simulink model "final_trust"  (R2014b)
settings: Solver=ode45  StartTime=0.0  StopTime=35  RelTol=1e-3
values from neighbouring files (symbols this model uses):
  adapt = 1    [init.m]    (also in init_model.m; init_mussels.m; init_mussels_2.m; init_mussels_konfiguracija_blizu.m)
  delta_0 = zeros(M,M)    [init_model.m]    (also in rander.m = zeros(n,1))
  K = 0.02    [init.m]    (also in init_model.m; init_mussels.m; init_mussels_2.m; init_mussels_konfiguracija_blizu.m)
  ko = ones(n,1)    [rander.m]
  n = input(prompt)    [init.m]    (also in init_consensus.m = 4; init_consensus_15.m = 15; init_mussels.m = 5; init_mussels_2.m = 5)
  sigma_0 = [ 0    0.7   0    0    0 ... (first row only)    [init.m]    (also in init_model.m = zeros(M,M); init_mussels.m = zeros(n,n); init_mussels_2.m; init_mussels_konfiguracija_blizu.m = [ 0    0.7   0.4    0.6    0.5)
  sko_x = transp(sko_x)    [fishplot.m]    (also in rander.m = [0.5, 1.5, 4, 4.5, 5, 7, 8, 9.5])
  sko_y = transp(sko_y)    [fishplot.m]    (also in rander.m = [8, 3, 5, 1, 4.5, 9, 3, 6])
  stream_x = [0.05,0.05,0.05,0.05]    [rander.m]
  stream_y = [0.03,0.03,0.03,0.03]    [rander.m]
  zeta_0 = zeros(n,n)    [init.m]    (also in init_model.m = zeros(M,M); init_mussels.m; init_mussels_2.m; init_mussels_konfiguracija_blizu.m)
undefined symbols (not defined in the file or in its folder): c_0, r, X, Y
settings Model: Creator=Demijan  LastModifiedBy=Demijan

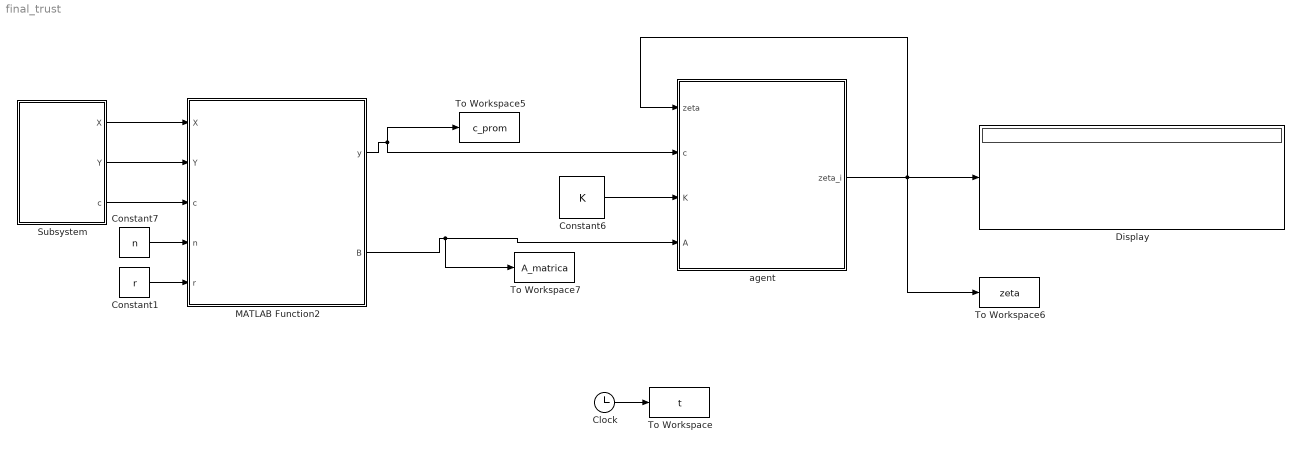
== system final_trust ==
  Clock : Clock
  Constant1 : Constant  Value=r
  Constant6 : Constant  Value=K
  Constant7 : Constant  Value=n
  Display : Display
  MATLAB Function2 : MATLAB Function  TreatAsAtomicUnit=on
  Subsystem : Subsystem
  To Workspace : ToWorkspace  VariableName=t  SampleTime=-1
  To Workspace5 : ToWorkspace  VariableName=c_prom  SampleTime=-1
  To Workspace6 : ToWorkspace  VariableName=zeta  SampleTime=-1
  To Workspace7 : ToWorkspace  VariableName=A_matrica  SampleTime=-1
  "agent " : Subsystem
  wires:
  Constant7/1 -> MATLAB Function2/4(n)
  Subsystem/3(c) -> MATLAB Function2/3(c)
  Subsystem/2(Y) -> MATLAB Function2/2(Y)
  Subsystem/1(X) -> MATLAB Function2/1(X)
  Constant6/1 -> "agent "/3(K)
  MATLAB Function2/1(y) -> "agent "/2(c), To Workspace5/1
  "agent "/1(zeta_i) -> Display/1, "agent "/1(zeta), To Workspace6/1
  Clock/1 -> To Workspace/1
  MATLAB Function2/2(B) -> "agent "/4(A), To Workspace7/1
  Constant1/1 -> MATLAB Function2/5(r)

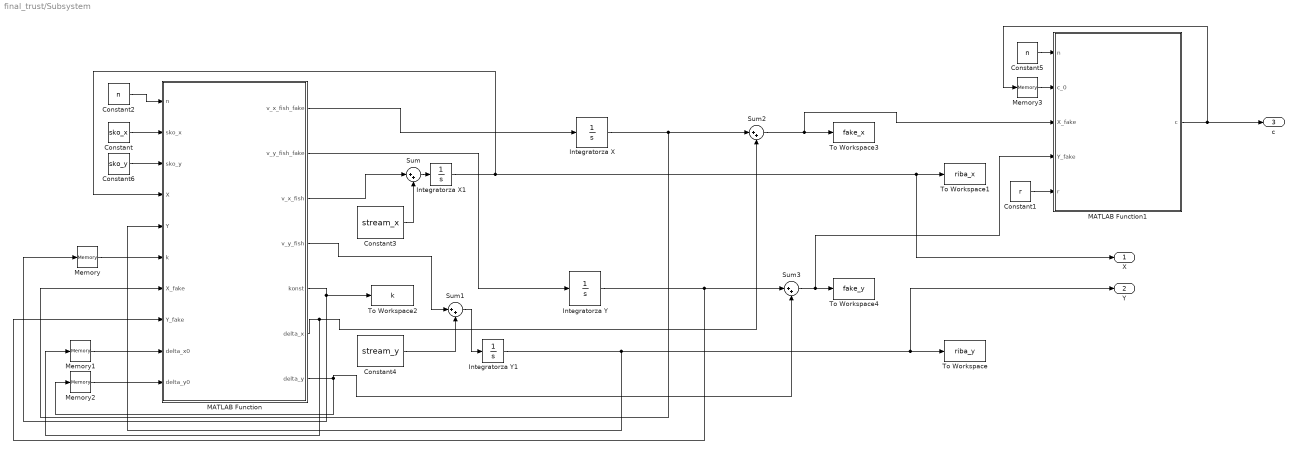
== system final_trust/Subsystem ==
  Constant : Constant  Value=sko_x
  Constant1 : Constant  Value=r
  Constant2 : Constant  Value=n
  Constant3 : Constant  Value=stream_x
  Constant4 : Constant  Value=stream_y
  Constant5 : Constant  Value=n
  Constant6 : Constant  Value=sko_y
  Integratorza X : Integrator  InitialCondition=X  LimitOutput=on  UpperSaturationLimit=10  LowerSaturationLimit=0
  Integratorza X1 : Integrator  InitialCondition=X  LimitOutput=on  UpperSaturationLimit=10  LowerSaturationLimit=0
  Integratorza Y : Integrator  InitialCondition=Y  LimitOutput=on  UpperSaturationLimit=10  LowerSaturationLimit=0
  Integratorza Y1 : Integrator  InitialCondition=Y  LimitOutput=on  UpperSaturationLimit=10  LowerSaturationLimit=0
  MATLAB Function : MATLAB Function  TreatAsAtomicUnit=on
  MATLAB Function1 : MATLAB Function  TreatAsAtomicUnit=on
  Memory : Memory  X0=ko  LinearizeAsDelay=on
  Memory1 : Memory  X0=delta_0  LinearizeAsDelay=on
  Memory2 : Memory  X0=delta_0  LinearizeAsDelay=on
  Memory3 : Memory  X0=c_0  LinearizeAsDelay=on
  Sum{,1..3} (4 alike) : Sum  Inputs=|++
  To Workspace : ToWorkspace  VariableName=riba_y  SaveFormat=Structure With Time  SampleTime=-1
  To Workspace1 : ToWorkspace  VariableName=riba_x  SaveFormat=Structure With Time  SampleTime=-1
  To Workspace2 : ToWorkspace  VariableName=k  SaveFormat=Structure With Time  SampleTime=-1
  To Workspace3 : ToWorkspace  VariableName=fake_x  SampleTime=-1
  To Workspace4 : ToWorkspace  VariableName=fake_y  SampleTime=-1
  X : Outport
  Y : Outport  Port=2
  c : Outport  Port=3
  wires:
  Constant2/1 -> MATLAB Function/1(n)
  Constant6/1 -> MATLAB Function/3(sko_y)
  Constant/1 -> MATLAB Function/2(sko_x)
  MATLAB Function/5(konst) -> To Workspace2/1, Memory/1
  Constant3/1 -> Sum/2
  Sum/1 -> Integratorza X1/1
  Constant4/1 -> Sum1/2
  Sum1/1 -> Integratorza Y1/1
  Integratorza Y1/1 -> MATLAB Function/5(Y), Y/1, To Workspace/1
  Integratorza X1/1 -> To Workspace1/1, X/1, MATLAB Function/4(X)
  Memory/1 -> MATLAB Function/6(k)
  MATLAB Function/6(delta_x) -> Memory1/1, Sum2/2
  MATLAB Function/7(delta_y) -> Sum3/2, Memory2/1
  Integratorza Y/1 -> MATLAB Function/8(Y_fake), Sum3/1
  Integratorza X/1 -> MATLAB Function/7(X_fake), Sum2/1
  Memory2/1 -> MATLAB Function/10(delta_y0)
  Memory1/1 -> MATLAB Function/9(delta_x0)
  MATLAB Function/1(v_x_fish_fake) -> Integratorza X/1
  MATLAB Function/3(v_x_fish) -> Sum/1
  MATLAB Function/4(v_y_fish) -> Sum1/1
  MATLAB Function/2(v_y_fish_fake) -> Integratorza Y/1
  Sum2/1 -> MATLAB Function1/3(X_fake), To Workspace3/1
  Sum3/1 -> MATLAB Function1/4(Y_fake), To Workspace4/1
  Constant1/1 -> MATLAB Function1/5(r)
  Constant5/1 -> MATLAB Function1/1(n)
  Memory3/1 -> MATLAB Function1/2(c_0)
  MATLAB Function1/1(c) -> Memory3/1, c/1

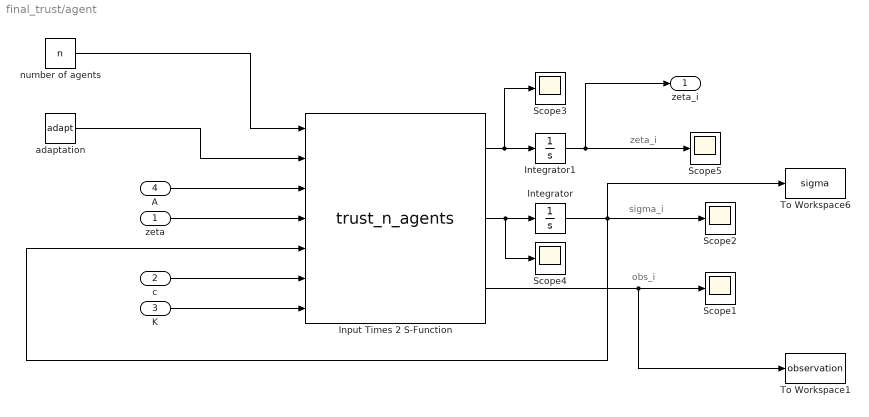
== system final_trust/agent  ==
  note: obs_i
  note: sigma_i
  note: zeta_i
  zeta : Inport
  c : Inport  Port=2
  K : Inport  Port=3
  A : Inport  Port=4
  Input Times 2 S-Function : S-Function  FunctionName=trust_n_agents  EnableBusSupport=off
  Integrator : Integrator  InitialCondition=sigma_0
  Integrator1 : Integrator  InitialCondition=zeta_0
  Scope{1..5} (5 alike) : Scope
      Scope1 settings: TimeRange=20  YMin=0.25  YMax=0.95
      Scope2 settings: TimeRange=20  YMin=0.25  YMax=0.95
      Scope3 settings: TimeRange=20  YMin=0.25  YMax=0.95  SaveName=ScopeData3
      Scope4 settings: TimeRange=20  YMin=0.25  YMax=0.95  SaveName=ScopeData4
      Scope5 settings: TimeRange=20  YMin=0.25  YMax=0.95  SaveName=ScopeData2
  To Workspace1 : ToWorkspace  VariableName=observation  SampleTime=-1
  To Workspace6 : ToWorkspace  VariableName=sigma  SampleTime=-1
  adaptation : Constant  Value=adapt
  number of agents : Constant  Value=n
  zeta_i : Outport
  wires:
  Integrator/1 -> Scope2/1, Input Times 2 S-Function/5, To Workspace6/1
  Integrator1/1 -> zeta_i/1, Scope5/1
  c/1 -> Input Times 2 S-Function/6
  K/1 -> Input Times 2 S-Function/7
  Input Times 2 S-Function/2 -> Scope4/1, Integrator/1
  Input Times 2 S-Function/1 -> Scope3/1, Integrator1/1
  Input Times 2 S-Function/3 -> To Workspace1/1, Scope1/1
  number of agents/1 -> Input Times 2 S-Function/1
  adaptation/1 -> Input Times 2 S-Function/2
  zeta/1 -> Input Times 2 S-Function/4
  A/1 -> Input Times 2 S-Function/3

== matlab function final_trust/MATLAB Function2 ==
  settings: updateMethod=DISCRETE  sampleTime=0.01
  data: y output; X input; Y input; c input; n input; B output; r input
function [y,B] = fish(X, Y, c, n, r)
A=zeros(20,20);
for i=1:n;
    for j=1:n;
        R = sqrt(((X(i)-X(j))^2+(Y(i)-Y(j))^2));
        if R < r && i~=j;
            A(i,j)=1;
        else
            A(i,j)=0;
        end
    end
end
B=zeros(4,4);
for i=1:n;
    for j=1:n;
        B(i,j)=A(i,j);
    end
end
y=zeros(4);
for i=1:n
  for j=1:n
      y(i,j)=A(i,j)*c(i,j);
  end
end

== matlab function final_trust/Subsystem/MATLAB Function ==
  data: v_x_fish_fake output; v_y_fish_fake output; n input; v_x_fish output; sko_x input; sko_y input; v_y_fish output; X input; Y input; k input; X_fake input; konst output; delta_x output; Y_fake input; delta_y output; delta_x0 input; delta_y0 input
function [v_x_fish_fake,v_y_fish_fake,v_x_fish,v_y_fish,konst,delta_x,delta_y] = fcn(n,sko_x, sko_y, X, Y,k,X_fake,Y_fake,delta_x0,delta_y0)
        d=[0; 0; 0; 0; 0; 0; 0; 0];        
        d_fake=[0; 0; 0; 0];
        red=zeros(4,8);
        red(1,:)=[1 3 1 2 3 2 1 3];
        red(2,:)=[2 3 1 3 1 3 1 2];
        red(3,:)=[2 3 2 3 1 3 2 1];
        red(4,:)=[2 1 2 3 2 3 1 3];
        d_x=[0; 0; 0; 0];
        d_y=[0; 0; 0; 0];
        v_x_fish=[0; 0; 0; 0];
        v_y_fish=[0; 0; 0; 0];
        d_x_fake=[0; 0; 0; 0];
        d_y_fake=[0; 0; 0; 0];
        v_x_fish_fake=[0; 0; 0; 0];
        v_y_fish_fake=[0; 0; 0; 0];
        delta_x=delta_x0;
        delta_y=delta_y0;
for i=1:n;
   d_x(i)=(sko_x(red(i,k(i)))-X(i));
   d_y(i)=(sko_y(red(i,k(i)))-Y(i));
   d_x_fake(i)=(sko_x(red(i,k(i)))-X_fake(i));
   d_y_fake(i)=(sko_y(red(i,k(i)))-Y_fake(i));
   d(i)=sqrt(d_x(i)^2+d_y(i)^2);
   d_fake(i)=sqrt(d_x_fake(i)^2+d_y_fake(i)^2);
   v_x_fish_fake(i)=(d_x_fake(i)/d_fake(i));
   v_y_fish_fake(i)=(d_y_fake(i)/d_fake(i));
   v_x_fish(i)=v_x_fish_fake(i);
   v_y_fish(i)=v_y_fish_fake(i);
   for j=1:4;
        if sqrt(((X(i)-sko_x(j))^2+(Y(i)-sko_y(j))^2))<=1;
           delta_x0(i)=X(i)-X_fake(i);
           delta_y0(i)=Y(i)-Y_fake(i);
           delta_x(i)=delta_x0(i);
           delta_y(i)=delta_y0(i);
           break;
        end
    end
    if(d(i)<=1);
       delta_x0(i)=X(i)-X_fake(i);
       delta_y0(i)=Y(i)-Y_fake(i);
       delta_x(i)=delta_x0(i);
       delta_y(i)=delta_y0(i);
       v_x_fish_fake(i)=0;
       v_y_fish_fake(i)=0;
       v_x_fish(i)=0;
       v_y_fish(i)=0;
       k(i)=k(i)+1;
       if(k(i)>=8);
           k(i)=1;
       end
    end
end
konst=k;
end

== matlab function final_trust/Subsystem/MATLAB Function1 ==
  data: c output; n input; c_0 input; X_fake input; Y_fake input; r input
function c  = fcn(n, c_0, X_fake,Y_fake,r) 
c=c_0;
for i=1:n;
   for j=1:n;
       c(i,j)=sqrt((X_fake(i)-X_fake(j))^2+(Y_fake(i)-Y_fake(j))^2)-r;
   end
end
end
